simulink model "example"  (R2022a)
settings: Solver=FixedStepAuto  StartTime=0.0  StopTime=inf  RelTol=1e-3
libraries: simulink x2, mttlib x1
settings Model: Creator=chrismailer  LastModifiedBy=chrismailer

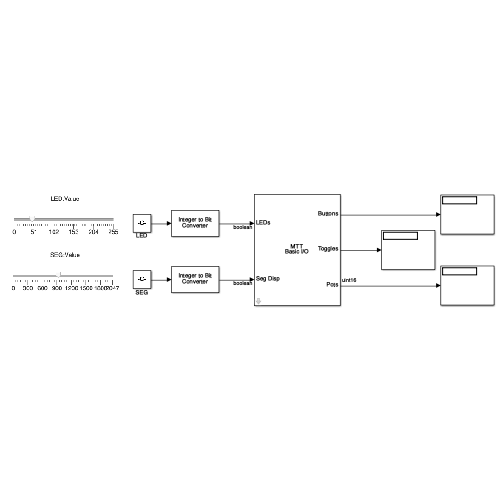
[thumbnail: Simulink's stored preview of the top-level diagram]
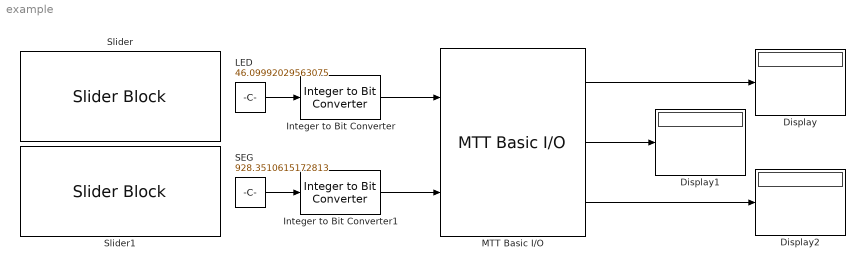
== system example ==
  Display : Display
  Display1 : Display
  Display2 : Display
  Integer to Bit Converter : simulink/Logic and Bit Operations/Integer to Bit Converter  nbits=8  signedInputValues=Unsigned  bitOrder=MSB first  outDtype=Inherit via internal rule
      settings: SourceProductBaseCode=SL
  Integer to Bit Converter1 : simulink/Logic and Bit Operations/Integer to Bit Converter  nbits=11  signedInputValues=Unsigned  bitOrder=MSB first  outDtype=Inherit via internal rule
      settings: SourceProductBaseCode=SL
  LED : Constant  Value=46.09992029563075  OutMin=[0]  OutMax=[255]  OutDataTypeStr=uint8
  MTT Basic I/O : mttlib/MTT Basic I//O  SelectedPort=/dev/cu.BLTH  SampleTime=0.01
  SEG : Constant  Value=928.3510615172813  OutMin=[0]  OutMax=[2047]  OutDataTypeStr=uint16
  Slider : SliderBlock  ScaleMax=255
  Slider1 : SliderBlock  ScaleMax=2047
  wires:
  MTT Basic I/O/1 -> Display/1
  MTT Basic I/O/2 -> Display1/1
  MTT Basic I/O/3 -> Display2/1
  Integer to Bit Converter/1 -> MTT Basic I/O/1
  LED/1 -> Integer to Bit Converter/1
  SEG/1 -> Integer to Bit Converter1/1
  Integer to Bit Converter1/1 -> MTT Basic I/O/2
